simulink model "vehicle_no_regulation"  (R2018a)
settings: Solver=ode23s  StartTime=0.0  StopTime=300  RelTol=1e-3
values from neighbouring files (symbols this model uses):
  B0 = 2.5    [init_params.m]
  Is = 0.2    [init_params.m]
  m = 100    [init_params.m]
  MFC1 = [9.5 1.9 1.14  0.75]    [init_params.m]
  MFC2 = [2.5 1.8 1 0.2]    [init_params.m]
  MFC3 = [1.5 1.8 0.4 0.2]    [init_params.m]
  N = 500    [init_params.m]
  r = 0.2    [init_params.m]
  v0 = 1    [init_params.m]
settings Model: Creator=obrusvit  LastModifiedBy=obrusvit

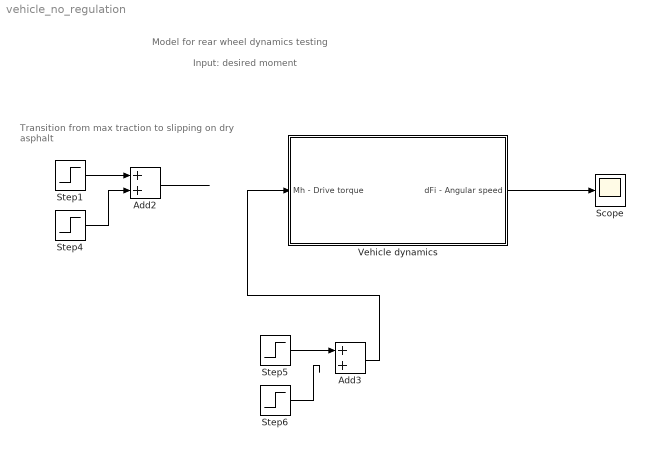
== system vehicle_no_regulation ==
  note: Input: desired moment
  note: Model for rear wheel dynamics testing
  note: Transition from max traction to slipping
      | on dry asphalt
  Add2 : Sum
  Add3 : Sum
  Scope : Scope
  Step1 : Step  Time=10  After=110  SampleTime=0
  Step4 : Step  Time=50  After=5  SampleTime=0
  Step5 : Step  Time=0  After=10  SampleTime=0
  Step6 : Step  Time=50  After=60  SampleTime=0
  Vehicle dynamics : Subsystem
  wires:
  Vehicle dynamics/1(dFi - Angular speed) -> Scope/1
  Add2/1 -> ?
  Step1/1 -> Add2/1
  Step4/1 -> Add2/2
  Step6/1 -> ?
  Step5/1 -> Add3/1
  Add3/1 -> Vehicle dynamics/1(Mh - Drive torque)

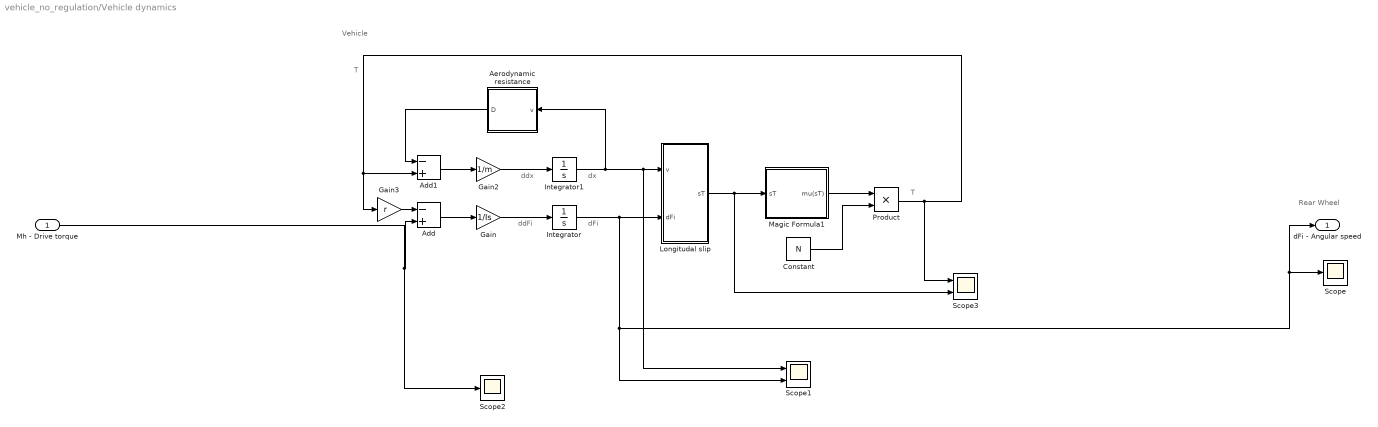
== system vehicle_no_regulation/Vehicle dynamics ==
  note: Vehicle
  note: Rear Wheel
  note: T
  note: ddx
  note: dx
  note: ddFi
  note: T
  note: dFi
  Mh - Drive torque : Inport
  Add : Sum  Inputs=-+
  Add1 : Sum  Inputs=-+
  "Aerodynamic resistance " : Subsystem
  Constant : Constant  Value=N
  Gain : Gain  Gain=1/Is
  Gain2 : Gain  Gain=1/m
  Gain3 : Gain  Gain=r
  Integrator : Integrator  InitialCondition=v0/r
  Integrator1 : Integrator  InitialCondition=v0
  Longitudal slip : Subsystem
  Magic Formula1 : Subsystem
  Product : Product
  Scope : Scope
  Scope1 : Scope  NumInputPorts=2
  Scope2 : Scope
  Scope3 : Scope  NumInputPorts=2
  dFi - Angular speed : Outport
  wires:
  Longitudal slip/1(sT) -> Magic Formula1/1(sT), Scope3/2
  Add1/1 -> Gain2/1
  Product/1 -> Gain3/1, Add1/2, Scope3/1
  Integrator1/1 -> "Aerodynamic resistance "/1(v), Scope1/1, Longitudal slip/1(v)
  "Aerodynamic resistance "/1("D ") -> Add1/1
  Gain3/1 -> Add/1
  Magic Formula1/1(mu(sT)) -> Product/1
  Gain/1 -> Integrator/1
  Add/1 -> Gain/1
  Mh - Drive torque/1 -> Scope2/1, Add/2
  Constant/1 -> Product/2
  Integrator/1 -> Scope1/2, dFi - Angular speed/1, Scope/1, Longitudal slip/2(dFi)
  Gain2/1 -> Integrator1/1

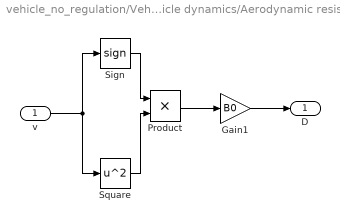
== system vehicle_no_regulation/Vehicle dynamics/Aerodynamic resistance  ==
  v : Inport
  Gain1 : Gain  Gain=B0
  Product : Product
  Sign : Signum
  Square : Math  Operator=square  SaturateOnIntegerOverflow=on
  "D " : Outport
  wires:
  v/1 -> Sign/1, Square/1
  Square/1 -> Product/2
  Sign/1 -> Product/1
  Gain1/1 -> "D "/1
  Product/1 -> Gain1/1

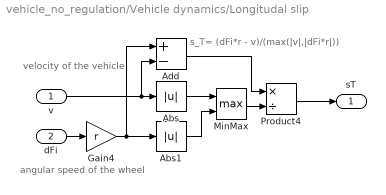
== system vehicle_no_regulation/Vehicle dynamics/Longitudal slip ==
  note: s_T= (dFi*r - v)/(max(|v|,|dFi*r|))
  note: angular speed
      | of the wheel
  note: velocity
      | of the vehicle
  v : Inport
  dFi : Inport  Port=2
  Abs : Abs
  Abs1 : Abs
  Add : Sum  Inputs=+-
  Gain4 : Gain  Gain=r
  MinMax : MinMax  Function=max  Inputs=2
  Product4 : Product  Inputs=*/  RndMeth=Zero
  sT : Outport
  wires:
  Product4/1 -> sT/1
  Add/1 -> Product4/1
  Abs1/1 -> MinMax/2
  Abs/1 -> MinMax/1
  MinMax/1 -> Product4/2
  Gain4/1 -> Add/1, Abs1/1
  dFi/1 -> Gain4/1
  v/1 -> Add/2, Abs/1

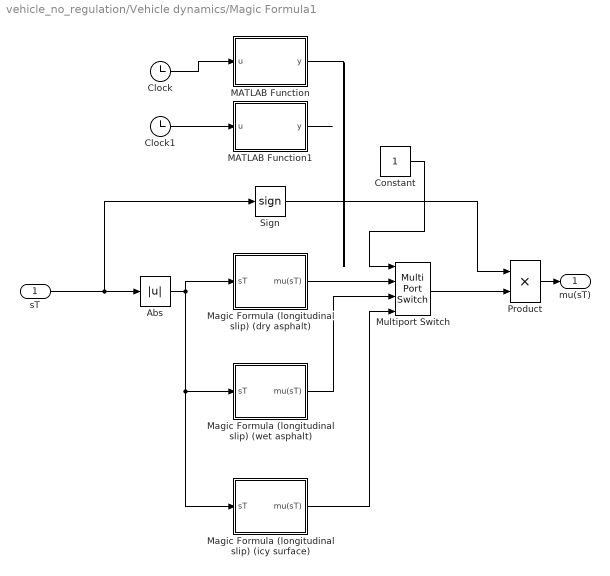
== system vehicle_no_regulation/Vehicle dynamics/Magic Formula1 ==
  sT : Inport
  Abs : Abs
  Clock : Clock
  Clock1 : Clock
  Constant : Constant
  MATLAB Function : MATLAB Function  TreatAsAtomicUnit=on
  MATLAB Function1 : MATLAB Function  TreatAsAtomicUnit=on
  Magic Formula (longitudinal slip) (dry asphalt) : Subsystem
  Magic Formula (longitudinal slip) (icy surface) : Subsystem
  Magic Formula (longitudinal slip) (wet asphalt) : Subsystem
  Multiport Switch : MultiPortSwitch
  Product : Product
  Sign : Signum
  mu(sT) : Outport
  wires:
  Abs/1 -> Magic Formula (longitudinal slip) (icy surface)/1(sT), Magic Formula (longitudinal slip) (wet asphalt)/1(sT), Magic Formula (longitudinal slip) (dry asphalt)/1(sT)
  Magic Formula (longitudinal slip) (dry asphalt)/1(mu(sT)) -> Multiport Switch/2
  Product/1 -> mu(sT)/1
  Sign/1 -> Product/1
  sT/1 -> Sign/1, Abs/1
  Magic Formula (longitudinal slip) (wet asphalt)/1(mu(sT)) -> Multiport Switch/3
  Multiport Switch/1 -> Product/2
  Magic Formula (longitudinal slip) (icy surface)/1(mu(sT)) -> Multiport Switch/4
  Clock/1 -> MATLAB Function/1(u)
  MATLAB Function/1(y) -> ?
  Constant/1 -> Multiport Switch/1
  Clock1/1 -> MATLAB Function1/1(u)
  MATLAB Function1/1(y) -> ?

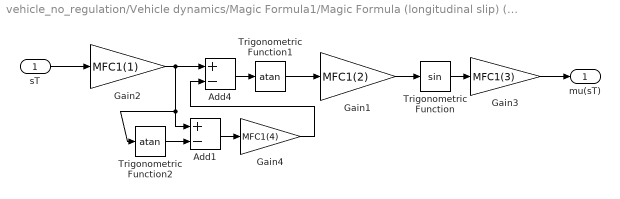
== system vehicle_no_regulation/Vehicle dynamics/Magic Formula1/Magic Formula (longitudinal slip) (dry asphalt) ==
  sT : Inport
  Add1 : Sum  Inputs=+-
  Add4 : Sum  Inputs=+-
  Gain1 : Gain  Gain=MFC1(2)
  Gain2 : Gain  Gain=MFC1(1)
  Gain3 : Gain  Gain=MFC1(3)
  Gain4 : Gain  Gain=MFC1(4)
  Trigonometric Function : Trigonometry
  Trigonometric Function1 : Trigonometry  Operator=atan
  Trigonometric Function2 : Trigonometry  Operator=atan
  mu(sT) : Outport
  wires:
  Gain3/1 -> mu(sT)/1
  sT/1 -> Gain2/1
  Add4/1 -> Trigonometric Function1/1
  Gain4/1 -> Add4/2
  Add1/1 -> Gain4/1
  Trigonometric Function2/1 -> Add1/2
  Gain2/1 -> Trigonometric Function2/1, Add1/1, Add4/1
  Trigonometric Function1/1 -> Gain1/1
  Gain1/1 -> Trigonometric Function/1
  Trigonometric Function/1 -> Gain3/1

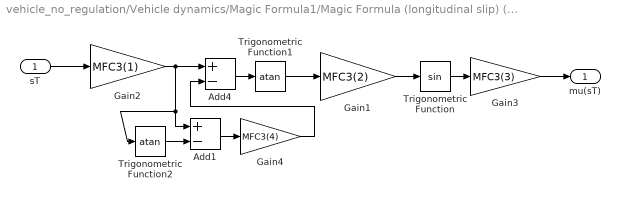
== system vehicle_no_regulation/Vehicle dynamics/Magic Formula1/Magic Formula (longitudinal slip) (icy surface) ==
  sT : Inport
  Add1 : Sum  Inputs=+-
  Add4 : Sum  Inputs=+-
  Gain1 : Gain  Gain=MFC3(2)
  Gain2 : Gain  Gain=MFC3(1)
  Gain3 : Gain  Gain=MFC3(3)
  Gain4 : Gain  Gain=MFC3(4)
  Trigonometric Function : Trigonometry
  Trigonometric Function1 : Trigonometry  Operator=atan
  Trigonometric Function2 : Trigonometry  Operator=atan
  mu(sT) : Outport
  wires:
  Gain3/1 -> mu(sT)/1
  sT/1 -> Gain2/1
  Add4/1 -> Trigonometric Function1/1
  Gain4/1 -> Add4/2
  Add1/1 -> Gain4/1
  Trigonometric Function2/1 -> Add1/2
  Gain2/1 -> Trigonometric Function2/1, Add1/1, Add4/1
  Trigonometric Function1/1 -> Gain1/1
  Gain1/1 -> Trigonometric Function/1
  Trigonometric Function/1 -> Gain3/1

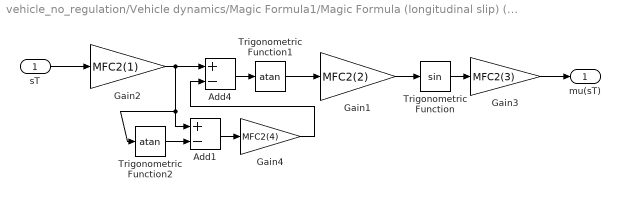
== system vehicle_no_regulation/Vehicle dynamics/Magic Formula1/Magic Formula (longitudinal slip) (wet asphalt) ==
  sT : Inport
  Add1 : Sum  Inputs=+-
  Add4 : Sum  Inputs=+-
  Gain1 : Gain  Gain=MFC2(2)
  Gain2 : Gain  Gain=MFC2(1)
  Gain3 : Gain  Gain=MFC2(3)
  Gain4 : Gain  Gain=MFC2(4)
  Trigonometric Function : Trigonometry
  Trigonometric Function1 : Trigonometry  Operator=atan
  Trigonometric Function2 : Trigonometry  Operator=atan
  mu(sT) : Outport
  wires:
  Gain3/1 -> mu(sT)/1
  sT/1 -> Gain2/1
  Add4/1 -> Trigonometric Function1/1
  Gain4/1 -> Add4/2
  Add1/1 -> Gain4/1
  Trigonometric Function2/1 -> Add1/2
  Gain2/1 -> Trigonometric Function2/1, Add1/1, Add4/1
  Trigonometric Function1/1 -> Gain1/1
  Gain1/1 -> Trigonometric Function/1
  Trigonometric Function/1 -> Gain3/1

== matlab function vehicle_no_regulation/Vehicle dynamics/Magic Formula1/MATLAB Function1 ==
  data: u input; y output
function y = fcn(u)
if u <= 150
    y = 3;
else
    y = 1;
end
end

== matlab function vehicle_no_regulation/Vehicle dynamics/Magic Formula1/MATLAB Function ==
  data: u input; y output
function y = fcn(u)
if u <= 20
    y = 1;
elseif u <= 40
    y = 2;
elseif u <= 60
    y = 3;
elseif u <= 80
    y = 2;
else
    y = 1;
end
end
